simulink model "Boucleouverte"  (R2017a)
settings: Solver=ode14x  StartTime=0.0  StopTime=800  FixedStep=0.01  RelTol=1e-3
values from neighbouring files (symbols this model uses):
  Parametres = [ax, bx, Rap, alpha, tau]    [Model.m]
  Parametres2 = [tr, f]    [Model.m]
settings Model: Creator=MONCEF  LastModifiedBy=MONCEF

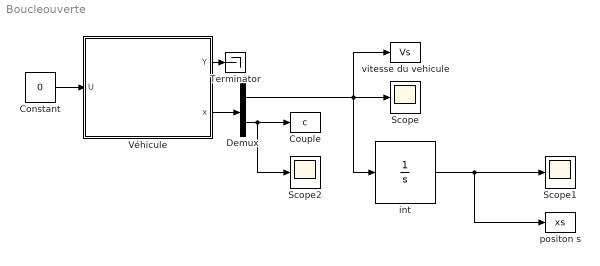
== system Boucleouverte ==
  Constant : Constant  Value=0
  Couple : ToWorkspace  VariableName=c  SaveFormat=Structure With Time  SampleTime=0.01
  Demux : Demux  Outputs=2
  Scope : Scope
  Scope1 : Scope
  Scope2 : Scope
  Terminator : Terminator
  Véhicule : Subsystem
      mask Display: image(fullfile(pwd,'Images','VehiculeSuiveur.jpg'));
  int : Integrator  InitialCondition=[1 1]
      mask Display: image(fullfile(pwd,'Images','Integrateur.png'));
  positon s : ToWorkspace  VariableName=xs  SaveFormat=Structure With Time  SampleTime=0.01
  vitesse du vehicule : ToWorkspace  VariableName=Vs  SaveFormat=Structure With Time  SampleTime=0.01
  wires:
  Véhicule/2(x) -> Demux/1
  Demux/1 -> vitesse du vehicule/1, Scope/1, int/1
  Demux/2 -> Couple/1, Scope2/1
  int/1 -> Scope1/1, positon s/1
  Véhicule/1(Y) -> Terminator/1
  Constant/1 -> Véhicule/1(U)

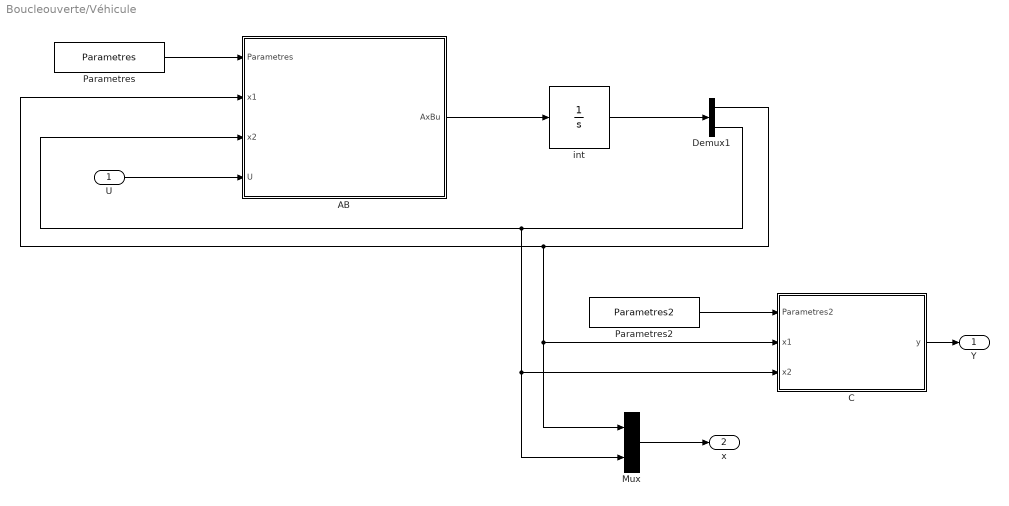
== system Boucleouverte/Véhicule ==
  U : Inport
  AB : MATLAB Function  TreatAsAtomicUnit=on
  C : MATLAB Function  TreatAsAtomicUnit=on
  Demux1 : Demux  Outputs=2
  Mux : Mux  Inputs=2
  Parametres : Constant  Value=Parametres
  Parametres2 : Constant  Value=Parametres2
  int : Integrator  InitialCondition=[10 0]
      mask Display: image(fullfile(pwd,'Images','Integrateur.png'));
  Y : Outport
  x : Outport  Port=2
  wires:
  C/1(y) -> Y/1
  Parametres/1 -> AB/1(Parametres)
  Parametres2/1 -> C/1(Parametres2)
  U/1 -> AB/4(U)
  AB/1(AxBu) -> int/1
  Demux1/2 -> Mux/2, C/3(x2), AB/3(x2)
  Demux1/1 -> Mux/1, C/2(x1), AB/2(x1)
  Mux/1 -> x/1
  int/1 -> Demux1/1

== matlab function Boucleouverte/Véhicule/AB ==
  data: Parametres input; x1 input; AxBu output; x2 input; U input
function AxBu = fcn(Parametres,x1,x2,U)

ax = Parametres(1);
bx = Parametres(2);
Rap = Parametres(3);
alpha = Parametres(4);
tau = Parametres(5);

%define the systeme matrix
A =[-(ax+bx*x1)/alpha Rap/alpha; 0 -1/tau];
B =[0 ; 1/tau];



AxBu = A*[x1;x2]+B*U;

== matlab function Boucleouverte/Véhicule/C ==
  data: Parametres2 input; x1 input; y output; x2 input
function y = fcn(Parametres2,x1,x2)
tr = Parametres2(1);
f = Parametres2(2);

C = [tr+f*x1 0];
y =C*[x1;x2];
